simulink model "simulacion_discreta"  (R2025a)
settings: Solver=VariableStepAuto  StartTime=0.0  StopTime=6  RelTol=1e-3
libraries: cstblocks x8
settings Model: Creator=danielsaenzobando  LastModifiedBy=danielsaenzobando

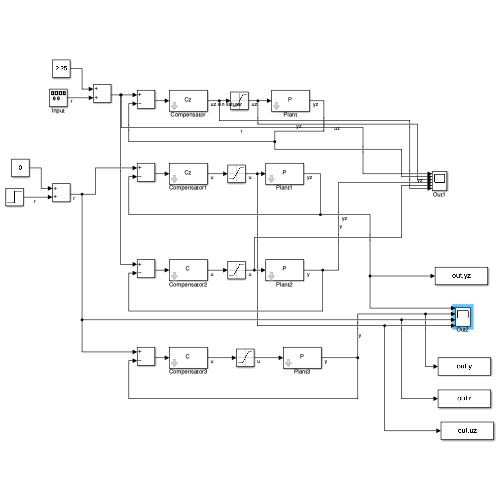
[thumbnail: Simulink's stored preview of the top-level diagram]
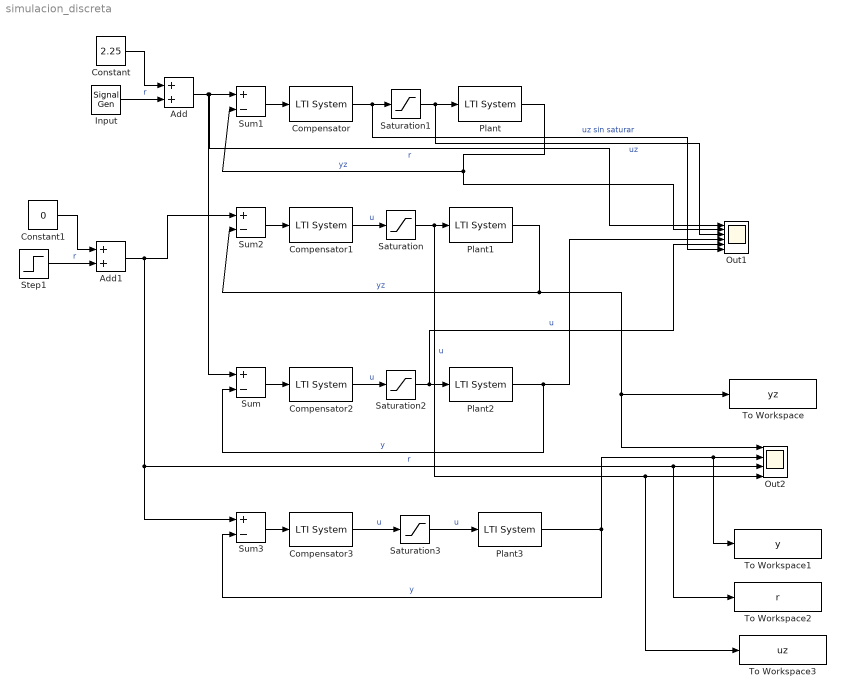
== system simulacion_discreta ==
  Add : Sum
  Add1 : Sum
  Compensator : cstblocks/LTI System  sys=Cz  IC=[]  PadeOrder=0
  Compensator1 : cstblocks/LTI System  sys=Cz  IC=[]  PadeOrder=0
  Compensator2 : cstblocks/LTI System  sys=C  IC=[]  PadeOrder=0
  Compensator3 : cstblocks/LTI System  sys=C  IC=[]  PadeOrder=0
  Constant : Constant  Value=2.25
  Constant1 : Constant  Value=0
  Input : SignalGenerator  WaveForm=square  Amplitude=1.25  Frequency=1/12
  Out1 : Scope  NumInputPorts=6
      settings: ActiveDisplayYMinimum=-2.37366085485109  ActiveDisplayYMaximum=6.81326009594375
  Out2 : Scope  NumInputPorts=4
      settings: ActiveDisplayYMinimum=-1  ActiveDisplayYMaximum=1
  Plant{,1..3} (4 alike) : cstblocks/LTI System  sys=P  IC=[]  PadeOrder=0
  Saturation{,1..3} (4 alike) : Saturate  UpperLimit=5  LowerLimit=0
  Step1 : Step  Time=0  SampleTime=0
  Sum{,1..3} (4 alike) : Sum  Inputs=+-
  To Workspace : ToWorkspace  VariableName=yz  SaveFormat=Timeseries  SampleTime=-1
  To Workspace1 : ToWorkspace  VariableName=y  SaveFormat=Timeseries  SampleTime=-1
  To Workspace2 : ToWorkspace  VariableName=r  SaveFormat=Timeseries  SampleTime=-1
  To Workspace3 : ToWorkspace  VariableName=uz  SaveFormat=Timeseries  SampleTime=-1
  wires:
  Sum1/1 -> Compensator/1
  Plant/1 -> Sum1/2, Out1/2  "yz"
  Input/1 -> Add/2  "r"
  Add/1 -> Out1/1, Sum1/1, Sum/1  "r"
  Constant/1 -> Add/1
  Sum2/1 -> Compensator1/1
  Plant1/1 -> Sum2/2, To Workspace/1, Out2/1  "yz"
  Plant2/1 -> Out1/4, Sum/2  "y"
  Plant3/1 -> To Workspace1/1, Out2/2, Sum3/2  "y"
  Sum/1 -> Compensator2/1
  Sum3/1 -> Compensator3/1
  Compensator1/1 -> Saturation/1  "u"
  Saturation/1 -> To Workspace3/1, Out2/4, Plant1/1  "u"
  Compensator/1 -> Out1/6, Saturation1/1  "uz sin saturar"
  Saturation1/1 -> Out1/3, Plant/1  "uz"
  Compensator2/1 -> Saturation2/1  "u"
  Saturation2/1 -> Out1/5, Plant2/1  "u"
  Compensator3/1 -> Saturation3/1  "u"
  Saturation3/1 -> Plant3/1  "u"
  Step1/1 -> Add1/2  "r"
  Constant1/1 -> Add1/1
  Add1/1 -> Sum3/1, To Workspace2/1, Out2/3, Sum2/1  "r"
